simulink model "hostModel_openLoop"  (R2023b)
settings: Solver=FixedStepDiscrete  StartTime=0.0  StopTime=inf  RelTol=1e-3  EnableMultiTasking=on
values from neighbouring files (symbols this model uses):
  PU_System = mcb_SetPUSystem(bldc,inverter)    [mcb_bldc_sixstep_f28069mLaunchPad_data.m]
  Ts = 0.03    [dataMonitoringArr.m]    (also in mcb_bldc_sixstep_f28069mLaunchPad_data.m = 5e-05)
libraries: instrumentseriallib x3, dspstat3 x3
settings Model: Creator=The MathWorks, Inc.  LastModifiedBy=Tefilus
settings SolverCC: AlgebraicLoopSolver=TrustRegion  MaxZcPerStep=1
settings DataIOCC: LimitDataPoints=on  SaveFormat=Array  ReturnWorkspaceOutputs=off
settings OptimizationCC: ReuseModelBlockBuffer=off  LifeSpan=1  EfficientTunableParamExpr=on
settings DebuggingCC: UnderspecifiedInitializationDetection=Classic  MergeDetectMultiDrivingBlocksExec=none  SolverPrmCheckMsg=warning  ParameterPrecisionLossMsg=none  UnconnectedInputMsg=warning  UnconnectedOutputMsg=warning  UnconnectedLineMsg=warning  AllowSymbolicDim=off  PregeneratedLibrarySubsystemCodeDiagnostic=none  SFUnexpectedBacktrackingDiag=warning  SFNoUnconditionalDefaultTransitionDiag=warning  SFExecutionAtInitializationDiag=none  ArithmeticOperatorsInVariantConditions=warning
settings HardwareCC: ProdBitPerPointer=32  ProdLargestAtomicFloat=None  ProdIntDivRoundTo=Undefined  ProdEndianess=Unspecified  ProdWordSize=32  ProdHWDeviceType=32-bit Generic
settings ModelReferenceCC: EnableRefExpFcnMdlSchedulingChecks=on  PropagateSignalLabelsOutOfModel=off
settings SFSimCC: SimUseLocalCustomCode=off  MATLABDynamicMemAlloc=off
settings RTWCC: Description=Real-Time Workshop Embedded Coder  SystemTargetFile=ert.tlc  TemplateMakefile=ert_default_tmf  GenerateReport=on  RTWUseLocalCustomCode=off  IncludeHyperlinkInReport=on  LaunchReport=on  GenerateTraceInfo=on  GenerateTraceReport=on  GenerateTraceReportSl=on  GenerateTraceReportSf=on  GenerateTraceReportEml=on  DLArmComputeVersion=19.05
settings CodeAppCC: IgnoreCustomStorageClasses=off  StateflowObjectComments=on  InternalIdentifier=Classic
settings ERTTargetCC: MultiwordLength=2048  GenerateSampleERTMain=on  ERTCustomFileTemplate=example_file_process.tlc  ConvertIfToSwitch=off  SuppressUnreachableDefaultCases=off
settings ConfigComp: CovMetricSettings=dw  CovSaveCumulativeToWorkspaceVar=on  CovSaveSingleToWorkspaceVar=on  CovExternalEMLEnable=off  CovSFcnEnable=off

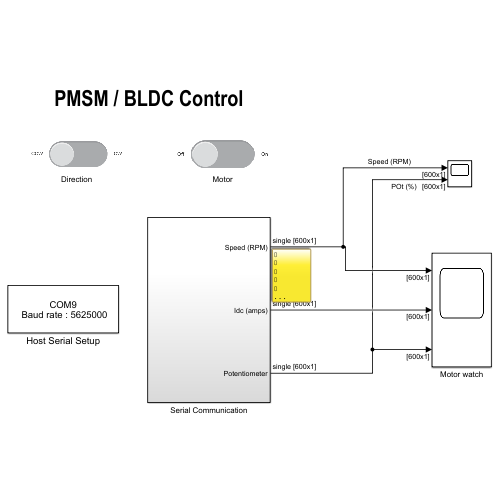
[thumbnail: Simulink's stored preview of the top-level diagram]
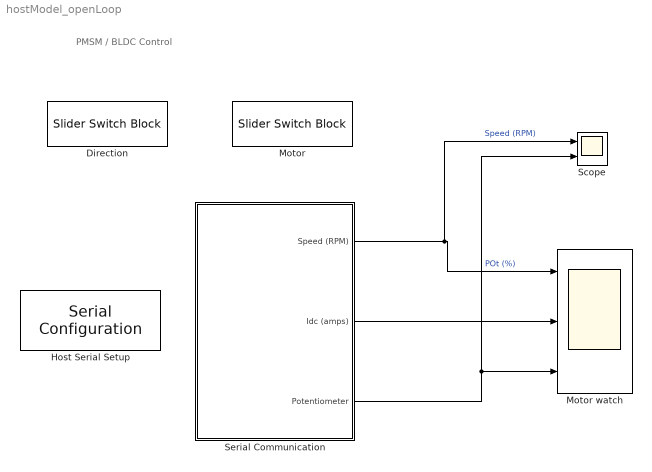
== system hostModel_openLoop ==
  note: PMSM / BLDC Control
  Direction : SliderSwitchBlock  LabelPosition=Hide
      settings: Values={{'CCW', 'CW'}, [0 1]}
  Host Serial Setup : instrumentseriallib/Serial Configuration  Priority=-99  PortSel=target.comport  Port=target.comport  ComPort=target.comport  BaudRate=5625000  DataBits=8  Parity=none  StopBits=1  ByteOrder=little-endian  FlowControl=none  Timeout=2  SimulateUsing=Interpreted execution  BlockInModel=on  aMode=5
  Motor : SliderSwitchBlock  LabelPosition=Hide
      settings: Values={{'Off', 'On'}, [0 1]}
  Motor watch : Scope  NumInputPorts=3
  Scope : Scope  NumInputPorts=2
  Serial Communication : Subsystem
  wires:
  Serial Communication/1(Speed (RPM)) -> Scope/1, Motor watch/1  "Speed (RPM)"
  Serial Communication/2(Idc (amps)) -> Motor watch/2
  Serial Communication/3(Potentiometer) -> Scope/2, Motor watch/3  "POt (%)"

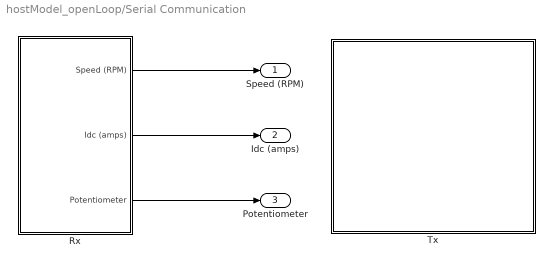
== system hostModel_openLoop/Serial Communication ==
  Rx : Subsystem
  Tx : Subsystem
  Speed (RPM) : Outport
  Idc (amps) : Outport  Port=2
  Potentiometer : Outport  Port=3
  wires:
  Rx/1(Speed (RPM)) -> Speed (RPM)/1
  Rx/2(Idc (amps)) -> Idc (amps)/1
  Rx/3(Potentiometer) -> Potentiometer/1

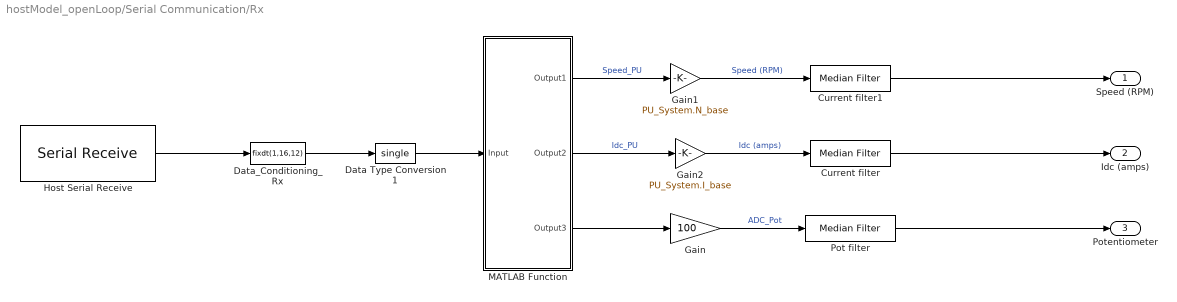
== system hostModel_openLoop/Serial Communication/Rx ==
  Current filter : dspstat3/Median Filter  WindowLength=5000  SimulateUsing=Interpreted execution
      settings: LibrarySourceBlock=|
      | dspfdesign/Median
      | Filter
  Current filter1 : dspstat3/Median Filter  WindowLength=5  SimulateUsing=Interpreted execution
      settings: LibrarySourceBlock=|
      | dspfdesign/Median
      | Filter
  Data Type Conversion1 : DataTypeConversion  OutDataTypeStr=single  RndMeth=Simplest  SaturateOnIntegerOverflow=off
  Data_Conditioning_Rx : DataTypeConversion  OutDataTypeStr=fixdt(1,16,12)  ConvertRealWorld=Stored Integer (SI)  RndMeth=Simplest  SaturateOnIntegerOverflow=off
  Gain : Gain  Gain=100
  Gain1 : Gain  Gain=PU_System.N_base  OutDataTypeStr=single  RndMeth=Simplest
  Gain2 : Gain  Gain=PU_System.I_base  OutDataTypeStr=single  RndMeth=Simplest
  Host Serial Receive : instrumentseriallib/Serial Receive  PortSel=target.comport  Port=target.comport  ComPort=target.comport  DataType=uint16  SaveDataType=uint8  ToggleHeader=on  Header='SS'  ToggleTerminator=on  Terminator=Custom terminator  CustomTerminator='EE'  InputFormat=Row major  ToggleDataSize=on  DataSize=[600 3]  EnableBlockingMode=on  ActionDataUnavailable=Output last received value  ActionWhenDataUnavailable=Output last received value  CustomValue=0  SampleTime=600 * Ts  SimulateUsing=Interpreted execution  BlockInModel=on  aMode=5
  MATLAB Function : MATLAB Function  TreatAsAtomicUnit=on
  Pot filter : dspstat3/Median Filter  WindowLength=5  SimulateUsing=Interpreted execution
      settings: LibrarySourceBlock=|
      | dspfdesign/Median
      | Filter
  Speed (RPM) : Outport
  Idc (amps) : Outport  Port=2
  Potentiometer : Outport  Port=3
  wires:
  MATLAB Function/3(Output3) -> Gain/1
  Data Type Conversion1/1 -> MATLAB Function/1(Input)
  Host Serial Receive/1 -> Data_Conditioning_Rx/1
  MATLAB Function/2(Output2) -> Gain2/1  "Idc_PU"
  MATLAB Function/1(Output1) -> Gain1/1  "Speed_PU"
  Gain1/1 -> Current filter1/1  "Speed (RPM)"
  Data_Conditioning_Rx/1 -> Data Type Conversion1/1
  Pot filter/1 -> Potentiometer/1
  Gain2/1 -> Current filter/1  "Idc (amps)"
  Gain/1 -> Pot filter/1  "ADC_Pot"
  Current filter1/1 -> Speed (RPM)/1
  Current filter/1 -> Idc (amps)/1

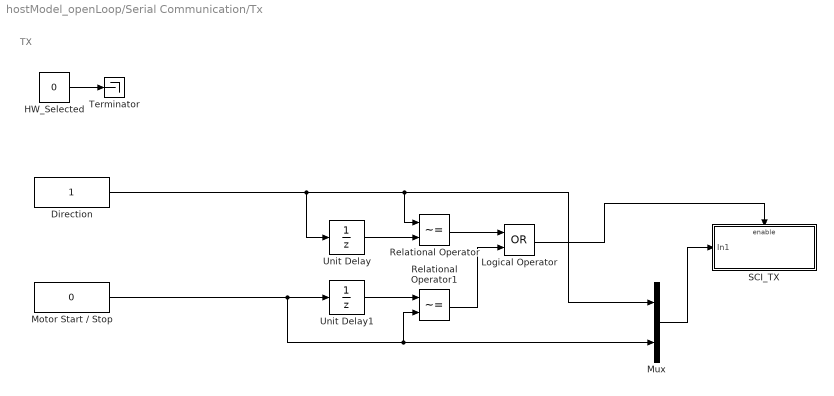
== system hostModel_openLoop/Serial Communication/Tx ==
  note: TX
  Direction : Constant  OutDataTypeStr=single
  HW_Selected : Constant  Value=0  OutDataTypeStr=uint8
  Logical Operator : Logic  Operator=OR  AllPortsSameDT=off  OutDataTypeStr=boolean
  Motor Start / Stop : Constant  Value=0  VectorParams1D=off  OutDataTypeStr=single
  Mux : Mux  Inputs=2
  Relational Operator : RelationalOperator  Operator=~=  OutDataTypeStr=boolean  InputSameDT=off
  Relational Operator1 : RelationalOperator  Operator=~=  OutDataTypeStr=boolean  InputSameDT=off
  SCI_TX : Subsystem  TreatAsAtomicUnit=on
  Terminator : Terminator
  Unit Delay : UnitDelay  SampleTime=-1  HasFrameUpgradeWarning=on
  Unit Delay1 : UnitDelay  SampleTime=-1  HasFrameUpgradeWarning=on
  wires:
  Motor Start / Stop/1 -> Relational Operator1/2, Mux/2, Unit Delay1/1
  HW_Selected/1 -> Terminator/1
  Relational Operator/1 -> Logical Operator/1
  Mux/1 -> SCI_TX/1(In1)
  Unit Delay/1 -> Relational Operator/2
  Unit Delay1/1 -> Relational Operator1/1
  Direction/1 -> Unit Delay/1, Mux/1, Relational Operator/1
  Logical Operator/1 -> SCI_TX/Enable
  Relational Operator1/1 -> Logical Operator/2

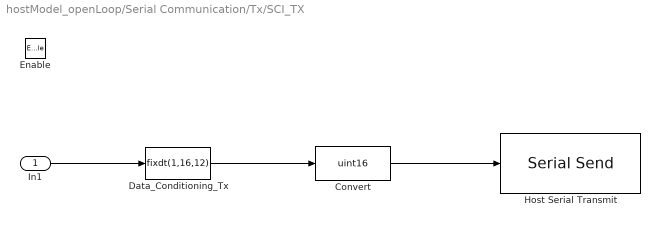
== system hostModel_openLoop/Serial Communication/Tx/SCI_TX ==
  In1 : Inport
  Enable : EnablePort
  Convert : DataTypeConversion  OutDataTypeStr=uint16  ConvertRealWorld=Stored Integer (SI)  RndMeth=Simplest  SaturateOnIntegerOverflow=off
  Data_Conditioning_Tx : DataTypeConversion  OutDataTypeStr=fixdt(1,16,12)  RndMeth=Simplest  SaturateOnIntegerOverflow=off
  Host Serial Transmit : instrumentseriallib/Serial Send  PortSel=target.comport  Port=target.comport  ComPort=target.comport  Header=[]  Terminator=<none>  CustomTerminator=[]  EnableBlockingMode=off  SimulateUsing=Interpreted execution  BlockInModel=on  aMode=5
  wires:
  Convert/1 -> Host Serial Transmit/1
  Data_Conditioning_Tx/1 -> Convert/1
  In1/1 -> Data_Conditioning_Tx/1

== matlab function hostModel_openLoop/Serial Communication/Rx/MATLAB Function ==
  data: Output1 output; Output2 output; Input input; Output3 output
 function [ Output1, Output2, Output3] = unBuf(Input)
Output1 = Input(:, 1);
Output2 = Input(:, 2);
Output3 = Input(:, 3);
end
